simulink model "torque_decompose"  (R2025b)
settings: Solver=FixedStepAuto  StartTime=0.0  StopTime=10.0  FixedStep=0.001  RelTol=1e-3
settings Model: Creator=lew11  LastModifiedBy=rosette-nebula

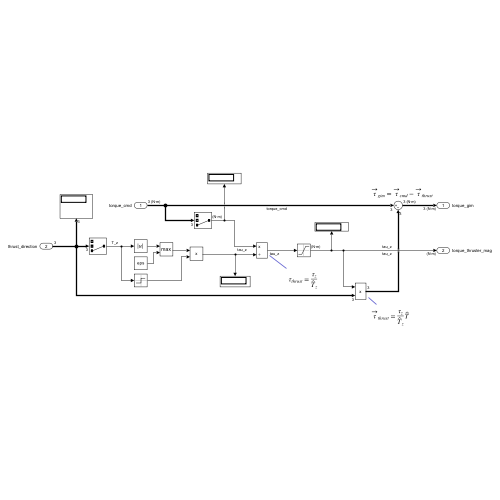
[thumbnail: Simulink's stored preview of the top-level diagram]
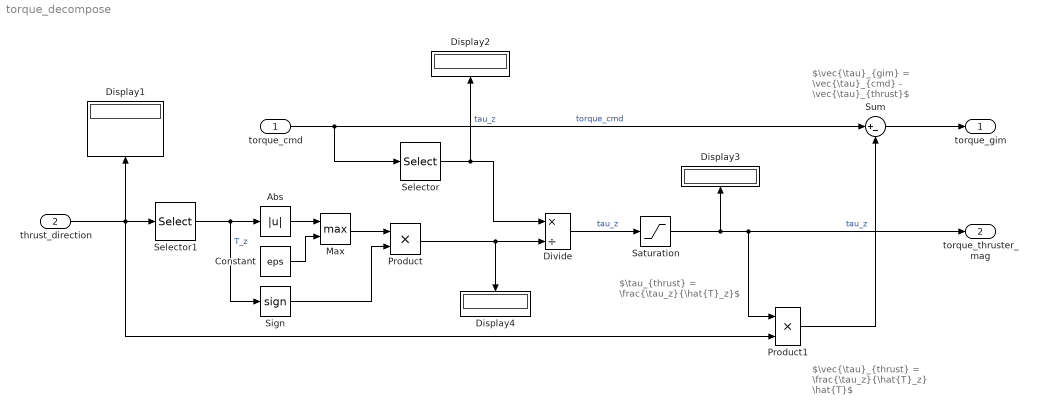
== system torque_decompose ==
  note: $\vec{\tau}_{thrust} = \frac{\tau_z}{\hat{T}_z} \hat{T}$
  note: $\tau_{thrust} = \frac{\tau_z}{\hat{T}_z}$
  note: $\vec{\tau}_{gim} = \vec{\tau}_{cmd} - \vec{\tau}_{thrust}$
  torque_cmd : Inport  Unit=N*m  PortDimensions=3
  thrust_direction : Inport  Port=2  PortDimensions=3
  Abs : Abs  SaturateOnIntegerOverflow=off
  Constant : Constant  Value=eps
  Display{1..4} (4 alike) : Display
  Divide : Product  Inputs=*/
  Max : MinMax  Function=max  Inputs=2
  Product : Product
  Product1 : Product
  Saturation : Saturate  UpperLimit=.45  LowerLimit=-.45
  Selector : Selector  InputPortWidth=3  IndexOptions=Index vector (dialog)  Indices=3  OutputSizes=1
  Selector1 : Selector  InputPortWidth=3  IndexOptions=Index vector (dialog)  Indices=3  OutputSizes=1
  Sign : Signum
  Sum : Sum  Inputs=|+-
  torque_gim : Outport  Unit=N*m  PortDimensions=3
  torque_thruster_mag : Outport  Port=2  Unit=N*m  PortDimensions=1
  wires:
  torque_cmd/1 -> Sum/1, Selector/1  "torque_cmd"
  thrust_direction/1 -> Product1/2, Display1/1, Selector1/1
  Selector/1 -> Display2/1, Divide/1  "tau_z"
  Sum/1 -> torque_gim/1
  Selector1/1 -> Sign/1, Abs/1  "T_z"
  Product1/1 -> Sum/2
  Product/1 -> Divide/2, Display4/1
  Divide/1 -> Saturation/1  "tau_z"
  Saturation/1 -> torque_thruster_mag/1, Product1/1, Display3/1  "tau_z"
  Abs/1 -> Max/1
  Constant/1 -> Max/2
  Sign/1 -> Product/2
  Max/1 -> Product/1
